simulink model "ControlSimulation"  (R2025b)
settings: Solver=VariableStepAuto  StartTime=0.0  StopTime=10.0  RelTol=1e-3
values from neighbouring files (symbols this model uses):
  A = simplify(A)    [LinModel.m]    (also in MainCtrl.m = A_reduced; MainCtrlSim.m = A_num; MainDyn.m = 50; MainObsv.m = A_reduced)
  B = simplify(hessian(K_total, dq))    [DDyn_Lagrange.m]    (also in DecompTau.m = sym(zeros(n)); ExtractInMat.m = sym(zeros(n)); LinModel.m = simplify(B); MainCtrl.m = B_reduced)
  C = simplify(C)    [LinModel.m]    (also in MainCtrl.m = C_reduced; MainCtrlSim.m = C_num; MainObsv.m = C_reduced)
undefined symbols (not defined in the file or in its folder): K
libraries: Robot_daVinci_Lib x1
settings Model: Creator=guilhermepifferchristo  LastModifiedBy=guilhermepifferchristo

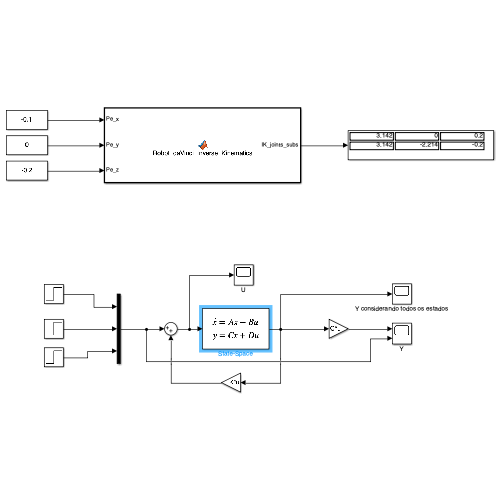
[thumbnail: Simulink's stored preview of the top-level diagram]
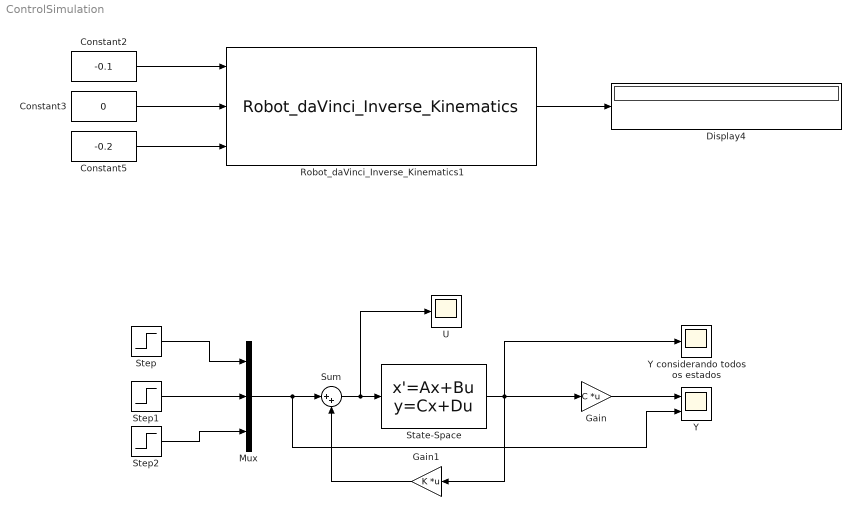
== system ControlSimulation ==
  Constant2 : Constant  Value=-0.1
  Constant3 : Constant  Value=0
  Constant5 : Constant  Value=-0.2
  Display4 : Display
  Gain : Gain  Gain=C  Multiplication=Matrix(K*u)
  Gain1 : Gain  Gain=K  Multiplication=Matrix(K*u)
  Mux : Mux  Inputs=3
  Robot_daVinci_Inverse_Kinematics1 : Robot_daVinci_Lib/Robot_daVinci_Inverse_Kinematics  SystemSampleTime=-1  VariantActivationTime=update diagram  EmptyChoice=off  PassThrough=off  PassThroughVariantControl=(default)  EmptyChoiceVariantControl=(default)  AllowFlexibleInterface=on  Latency=0  AutoFrameSizeCalculation=off
  State-Space : StateSpace  A=A  B=B  C=eye(5)  D=zeros(5,3)  InitialCondition=0
  Step : Step  SampleTime=0
  Step1 : Step  SampleTime=0
  Step2 : Step  SampleTime=0
  Sum : Sum  Inputs=|++
  U : Scope
      settings: DataLoggingVariableName=ScopeData2
  Y : Scope  NumInputPorts=2
      settings: ActiveDisplayYMinimum=-0.13092052421091982  ActiveDisplayYMaximum=1.1782847178982787
  Y considerando todos os estados : Scope
      settings: ActiveDisplayYMinimum=-0.18068159377472626  ActiveDisplayYMaximum=1.1834049103746023
  wires:
  Step/1 -> Mux/1
  Mux/1 -> Y/2, Sum/1
  Step1/1 -> Mux/2
  Step2/1 -> Mux/3
  Sum/1 -> U/1, State-Space/1
  Constant5/1 -> Robot_daVinci_Inverse_Kinematics1/3
  Constant2/1 -> Robot_daVinci_Inverse_Kinematics1/1
  Constant3/1 -> Robot_daVinci_Inverse_Kinematics1/2
  Robot_daVinci_Inverse_Kinematics1/1 -> Display4/1
  State-Space/1 -> Y considerando todos os estados/1, Gain1/1, Gain/1
  Gain/1 -> Y/1
  Gain1/1 -> Sum/2
